simulink model "LQR_6DoF_v4"  (R2022b)
settings: Solver=ode45  StartTime=0.0  StopTime=10  FixedStep=0.01  RelTol=1e-3
undefined symbols (not defined in the file): beta, e0_0, e1_0, e2_0, e3_0, eul0, G0, gamma, gc, geometry, Js, Js0, K_lqrq, m_dry, m_fuel, m_full, m_max, mass, omega0, parameters, pos0, r_cg, rcgs, ref_eul, Tensors, vel0, xq0
libraries: sharedtransform x38, simulink_extras x21, matrix_library x12, sharedutil x4, aerolibpropulsion2 x1
(part 2 of 2)

== system LQR_6DoF_v4/NL Custom Model with Quaternions/Initial Conditions ==
  Constant2 : Constant  Value=omega0
  Initial Euler Angles : Constant  Value=eul0
  Initial Position : Constant  Value=pos0
  Initial velocity : Constant  Value=vel0
  Mux : Mux
  Rotation Angles to Quaternions : sharedtransform/Rotation Angles to Quaternions  rotationOrder=ZYX  aMode=aMode
      settings: LibrarySourceBlock=shared6dofsys/DCM & Euler Angles (Quaternion)/Rotation Angles to Quaternions
  Selector : Selector  InputPortWidth=3  IndexOptions=Index vector (dialog)  Indices=[2 3 1]  OutputSizes=1
  x0 : Outport
  wires:
  Rotation Angles to Quaternions/1 -> Mux/3
  Constant2/1 -> Mux/4
  Initial Position/1 -> Mux/1
  Selector/1 -> Rotation Angles to Quaternions/1
  Initial Euler Angles/1 -> Selector/1
  Initial velocity/1 -> Mux/2
  Mux/1 -> x0/1

== system LQR_6DoF_v4/NL Custom Model with Quaternions/Quaternion2DCM ==
  q : Inport
  A11 : sharedtransform/Quaternions to  Direction Cosine Matrix/A11  SystemSampleTime=-1  VariantActivationTime=update diagram  Latency=0  AutoFrameSizeCalculation=off
  A12 : sharedtransform/Quaternions to  Direction Cosine Matrix/A12  SystemSampleTime=-1  VariantActivationTime=update diagram  Latency=0  AutoFrameSizeCalculation=off
  A13 : sharedtransform/Quaternions to  Direction Cosine Matrix/A13  SystemSampleTime=-1  VariantActivationTime=update diagram  Latency=0  AutoFrameSizeCalculation=off
  A21 : sharedtransform/Quaternions to  Direction Cosine Matrix/A21  SystemSampleTime=-1  VariantActivationTime=update diagram  Latency=0  AutoFrameSizeCalculation=off
  A22 : sharedtransform/Quaternions to  Direction Cosine Matrix/A22  SystemSampleTime=-1  VariantActivationTime=update diagram  Latency=0  AutoFrameSizeCalculation=off
  A23 : sharedtransform/Quaternions to  Direction Cosine Matrix/A23  SystemSampleTime=-1  VariantActivationTime=update diagram  Latency=0  AutoFrameSizeCalculation=off
  A31 : sharedtransform/Quaternions to  Direction Cosine Matrix/A31  SystemSampleTime=-1  VariantActivationTime=update diagram  Latency=0  AutoFrameSizeCalculation=off
  A32 : sharedtransform/Quaternions to  Direction Cosine Matrix/A32  SystemSampleTime=-1  VariantActivationTime=update diagram  Latency=0  AutoFrameSizeCalculation=off
  A33 : sharedtransform/Quaternions to  Direction Cosine Matrix/A33  SystemSampleTime=-1  VariantActivationTime=update diagram  Latency=0  AutoFrameSizeCalculation=off
  Create 3x3 Matrix : sharedutil/Create 3x3 Matrix  aMode=aMode
  Quaternion Normalize : sharedutil/Quaternion Normalize  aMode=aMode
  DCMq : Outport
  wires:
  A12/1 -> Create 3x3 Matrix/2
  A13/1 -> Create 3x3 Matrix/3
  Quaternion Normalize/1 -> A11/1, A12/1, A13/1, A21/1, A22/1, A23/1, A31/1, A32/1, A33/1
  A21/1 -> Create 3x3 Matrix/4
  A33/1 -> Create 3x3 Matrix/9
  A22/1 -> Create 3x3 Matrix/5
  A31/1 -> Create 3x3 Matrix/7
  A11/1 -> Create 3x3 Matrix/1
  A23/1 -> Create 3x3 Matrix/6
  A32/1 -> Create 3x3 Matrix/8
  Create 3x3 Matrix/1 -> DCMq/1
  q/1 -> Quaternion Normalize/1

== system LQR_6DoF_v4/6DOF HopperDynamic/Rocket Dynamics 6DOF2/Calculate DCM & Euler Angles ==
  p q r : Inport
  Display : Display
  Display1 : Display
  Initial Euler Angles : Constant  Value=eul_0
  Quaternions to Direction Cosine Matrix : sharedtransform/Quaternions to  Direction Cosine Matrix  aMode=aMode
  Quaternions to Rotation Angles : sharedtransform/Quaternions to Rotation Angles  rotationOrder=ZYX  aMode=aMode
  Rotation Angles to Direction Cosine Matrix1 : sharedtransform/Rotation Angles to Direction Cosine Matrix  rotationOrder=ZYX  aMode=aMode
  Rotation Angles to Quaternions : sharedtransform/Rotation Angles to Quaternions  rotationOrder=ZYX  aMode=aMode
  Selector : Selector  InputPortWidth=3  IndexOptions=Index vector (dialog)  Indices=[3 1 2]  OutputSizes=1
  Selector1 : Selector  InputPortWidth=3  IndexOptions=Index vector (dialog)  Indices=[2 3 1]  OutputSizes=1
  Selector2 : Selector  InputPortWidth=3  IndexOptions=Index vector (dialog)  Indices=[2 3 1]  OutputSizes=1
  Terminator1 : Terminator
  phi theta psi : Integrator  InitialConditionSource=external  InitialCondition=[0, pi/2, 0]  WrapState=on
  phi_dot theta_dot psi_dot : Subsystem
  q0 q1 q2 q3 : Integrator  InitialConditionSource=external  InitialCondition=[e0_0 e1_0 e2_0 e3_0]  ContinuousStateAttributes=quat_statename
  qdot : Subsystem
  DCM : Outport  VectorParamsAs1DForOutWhenUnconnected=off
  Euler : Outport  Port=2  VectorParamsAs1DForOutWhenUnconnected=off
  Quaternion : Outport  Port=3
  wires:
  Selector1/1 -> Rotation Angles to Quaternions/1
  qdot/1(qdot) -> q0 q1 q2 q3/1
  p q r/1 -> phi_dot theta_dot psi_dot/1(p q r), qdot/1(p q r)
  Quaternions to Direction Cosine Matrix/1 -> Display/1, DCM/1
  Rotation Angles to Quaternions/1 -> q0 q1 q2 q3/2
  Quaternions to Rotation Angles/1 -> Selector/1
  Selector/1 -> Terminator1/1
  q0 q1 q2 q3/1 -> Quaternion/1, qdot/2(q0 q1 q2 q3), Quaternions to Rotation Angles/1, Quaternions to Direction Cosine Matrix/1
  phi_dot theta_dot psi_dot/1(phidot thetadot psidot) -> phi theta psi/1
  Selector2/1 -> Rotation Angles to Direction Cosine Matrix1/1
  Initial Euler Angles/1 -> phi theta psi/2, Selector1/1
  Rotation Angles to Direction Cosine Matrix1/1 -> Display1/1
  phi theta psi/1 -> Euler/1, Selector2/1, phi_dot theta_dot psi_dot/2(phi theta psi)

== system LQR_6DoF_v4/6DOF HopperDynamic/Rocket Dynamics 6DOF2/Calculate omega_dot ==
  p q r : Inport
  "I, I_dot" : Inport  Port=2
  Moments : Inport  Port=3
  3x3 Cross Product : sharedutil/3x3 Cross Product  aMode=aMode
  I x w : Subsystem
  I x w1 : Subsystem
  Product2 : Product  Inputs=*/  Multiplication=Matrix(*)  SaturateOnIntegerOverflow=on  OutDataTypeStr=Inherit: Same as first input
  Reshape : Reshape
  Reshape1 : Reshape  OutputDimensionality=Row vector (2-D)
  Selector : Selector  NumberOfDimensions=2  InputPortWidth=2  IndexOptions=Index vector (dialog),Select all  Indices=1:3,-1  OutputSizes=1
  Selector1 : Selector  NumberOfDimensions=2  InputPortWidth=2  IndexOptions=Index vector (dialog),Select all  Indices=4:6,-1  OutputSizes=1
  Selector2 : Selector  NumberOfDimensions=2  InputPortWidth=2  IndexOptions=Index vector (dialog),Select all  Indices=1:3,-1  OutputSizes=1
  Sum2 : Sum  Inputs=+--  SaturateOnIntegerOverflow=on
  pdot qdot rdot : Outport  VectorParamsAs1DForOutWhenUnconnected=off
  wires:
  "I, I_dot"/1 -> Selector1/1, Selector2/1, Selector/1
  Selector/1 -> I x w/2(Inertia)
  I x w/1(I * w) -> 3x3 Cross Product/2
  p q r/1 -> I x w1/2(p q r), 3x3 Cross Product/1, I x w/1(p q r)
  Moments/1 -> Sum2/1
  I x w1/1(Id * w) -> Sum2/2
  3x3 Cross Product/1 -> Sum2/3
  Sum2/1 -> Reshape1/1
  Reshape/1 -> pdot qdot rdot/1
  Selector2/1 -> Product2/2
  Reshape1/1 -> Product2/1
  Product2/1 -> Reshape/1
  Selector1/1 -> I x w1/1(I_dot)

== system LQR_6DoF_v4/6DOF HopperDynamic/Rocket Dynamics 6DOF2/Determine Force, Mass & Inertia ==
  forces : Inport
  "mass " : Inport  Port=2
  I : Inport  Port=3
  I_dot : Inport  Port=4
  Matrix Concatenation : Concatenate  Mode=Multidimensional array
  "forces " : Outport  PortDimensions=3  VectorParamsAs1DForOutWhenUnconnected=off
  mass : Outport  Port=2  VectorParamsAs1DForOutWhenUnconnected=off
  "I, I_dot " : Outport  Port=3  VectorParamsAs1DForOutWhenUnconnected=off
  wires:
  "mass "/1 -> mass/1
  I/1 -> Matrix Concatenation/1
  I_dot/1 -> Matrix Concatenation/2
  Matrix Concatenation/1 -> "I, I_dot "/1
  forces/1 -> "forces "/1

== system LQR_6DoF_v4/6DOF HopperDynamic/Rocket Dynamics 6DOF2/transform to Inertial axes ==
  x y z : Inport
  transform coefficients : Inport  Port=2
  Product : Product  Multiplication=Matrix(*)  InputSameDT=on  SaturateOnIntegerOverflow=on  OutDataTypeStr=Inherit: Same as first input
  Reshape1 : Reshape  OutputDimensionality=Column vector (2-D)
  Reshape2 : Reshape
  Ve : Outport  VectorParamsAs1DForOutWhenUnconnected=off
  wires:
  transform coefficients/1 -> Product/1
  Product/1 -> Reshape2/1
  Reshape1/1 -> Product/2
  x y z/1 -> Reshape1/1
  Reshape2/1 -> Ve/1

== system LQR_6DoF_v4/6DOF HopperDynamic/Rocket Dynamics 6DOF2/Calculate DCM & Euler Angles/phi_dot theta_dot psi_dot ==
  p q r : Inport
  phi theta psi : Inport  Port=2
  Mux1 : Mux  Inputs=[3 3 3]
  Mux2 : Mux  Inputs=3
  phi psi theta : Selector  InputPortWidth=3  IndexOptions=Index vector (dialog)  Indices=[1 3 2]  OutputSizes=1
  phidot : Fcn  Expr=u[1]+(u[2]*u[4]+u[3]*u[7])*(u[5]/u[8])
  psidot : Fcn  Expr=u[2]*u[7]-u[3]*u[4]
  sincos : Trigonometry  Operator=sincos
  thetadot : Fcn  Expr=(u[2]*u[4]+u[3]*u[7])/u[8]
  phidot thetadot psidot : Outport
  wires:
  phidot/1 -> Mux2/1
  thetadot/1 -> Mux2/2
  sincos/1 -> Mux1/2
  Mux1/1 -> psidot/1, thetadot/1, phidot/1
  p q r/1 -> Mux1/1
  sincos/2 -> Mux1/3
  psidot/1 -> Mux2/3
  phi theta psi/1 -> phi psi theta/1
  phi psi theta/1 -> sincos/1
  Mux2/1 -> phidot thetadot psidot/1

== system LQR_6DoF_v4/6DOF HopperDynamic/Rocket Dynamics 6DOF2/Calculate DCM & Euler Angles/qdot ==
  p q r : Inport
  q0 q1 q2 q3 : Inport  Port=2
  Constant : Constant
  Dot Product : DotProduct  InputSameDT=off  OutDataTypeStr=Inherit: Inherit via internal rule
  High Gain Quaternion Normalization : Gain  Gain=k_quat  SaturateOnIntegerOverflow=on  OutDataTypeStr=Inherit: Same as input  ParamDataTypeStr=Inherit: Same as input
  Mux1 : Mux  Inputs=[3 4 1]
  Mux2 : Mux
  Sum : Sum  Inputs=|+-  InputSameDT=on  SaturateOnIntegerOverflow=on  OutDataTypeStr=Inherit: Same as first input
  q0dot : Fcn  Expr=-0.5 * ( u[5]*u[1]+u[6]*u[2]+u[7]*u[3] ) + u[8]*u[4]
  q1dot : Fcn  Expr=0.5 * ( u[4]*u[1]+u[6]*u[3]-u[7]*u[2] ) + u[8]*u[5]
  q2dot : Fcn  Expr=0.5 * ( u[4]*u[2]+u[7]*u[1]-u[5]*u[3] ) + u[8]*u[6]
  q3dot : Fcn  Expr=0.5 * ( u[4]*u[3]+u[5]*u[2]-u[6]*u[1] ) + u[8]*u[7]
  qdot : Outport  InitialOutput=0  VectorParamsAs1DForOutWhenUnconnected=off
  wires:
  q0dot/1 -> Mux2/1
  Sum/1 -> High Gain Quaternion Normalization/1
  Constant/1 -> Sum/1
  p q r/1 -> Mux1/1
  High Gain Quaternion Normalization/1 -> Mux1/3
  Dot Product/1 -> Sum/2
  q0 q1 q2 q3/1 -> Dot Product/1, Dot Product/2, Mux1/2
  Mux2/1 -> qdot/1
  q3dot/1 -> Mux2/4
  Mux1/1 -> q2dot/1, q3dot/1, q0dot/1, q1dot/1
  q2dot/1 -> Mux2/3
  q1dot/1 -> Mux2/2

== system LQR_6DoF_v4/6DOF HopperDynamic/Rocket Dynamics 6DOF2/Calculate omega_dot/I x w ==
  p q r : Inport
  Inertia : Inport  Port=2
  Product : Product  Multiplication=Matrix(*)  InputSameDT=on  SaturateOnIntegerOverflow=on  OutDataTypeStr=Inherit: Same as first input
  Reshape1 : Reshape  OutputDimensionality=Column vector (2-D)
  Reshape2 : Reshape
  I * w : Outport  VectorParamsAs1DForOutWhenUnconnected=off
  wires:
  Inertia/1 -> Product/1
  Reshape1/1 -> Product/2
  Product/1 -> Reshape2/1
  p q r/1 -> Reshape1/1
  Reshape2/1 -> I * w/1

== system LQR_6DoF_v4/6DOF HopperDynamic/Rocket Dynamics 6DOF2/Calculate omega_dot/I x w1 ==
  I_dot : Inport
  p q r : Inport  Port=2
  Product : Product  Multiplication=Matrix(*)  InputSameDT=on  SaturateOnIntegerOverflow=on  OutDataTypeStr=Inherit: Same as first input
  Reshape1 : Reshape  OutputDimensionality=Column vector (2-D)
  Reshape2 : Reshape
  Id * w : Outport  VectorParamsAs1DForOutWhenUnconnected=off
  wires:
  I_dot/1 -> Product/1
  Reshape1/1 -> Product/2
  Product/1 -> Reshape2/1
  p q r/1 -> Reshape1/1
  Reshape2/1 -> Id * w/1

== matlab function LQR_6DoF_v4/Actuator Forces/Center of Mass1 ==
  data: m_input input; CoM output; mass input; rcgs input
function CoM = current_CoM(m_input, mass, rcgs)
    CoM = mass_center_interpolate(m_input, mass, rcgs);

== matlab function LQR_6DoF_v4/6DOF HopperDynamic/MATLAB Function ==
  data: m_current input; J output; mass input; Tensors input
function J = Tensor_of_Inertia(m_current, mass, Tensors)
    % interpolation components of tensor of inertia
    J = tensor_interpolation(m_current, mass, Tensors);
end

== matlab function LQR_6DoF_v4/NL Custom Model with Quaternions/MATLAB Function ==
  data: t input; x input; u input; xdot output; Jo input; Jdot input; m input; DCM_e output; G output; p input
function [xdot, DCM_e, G] = NL_HopperDyn(t, x, u, Jo, Jdot, m, p)
    % for debuging
    if t > 10.4
        i = 10;
    end
    [xdot, DCM_e, G] = NL_HopperDyn_v3_quat(x, u, Jo, Jdot, m, p, [0;0;0;0;0;0]);
